simulink model "sim_sistema_2"  (Simulink 7.5)
settings: Solver=ode3  StartTime=0.0  StopTime=10  FixedStep=1e-4  RelTol=1e-3
values from neighbouring files (symbols this model uses):
  K = acker(sis.a,sis.b,J)    [sistema_2.m]    (also in sistema_2_observador.m)
  sis = ss(sis)    [sistema_2.m]    (also in sistema_2_observador.m)
settings Model: Creator=taniel.franklin  LastModifiedBy=taniel.franklin

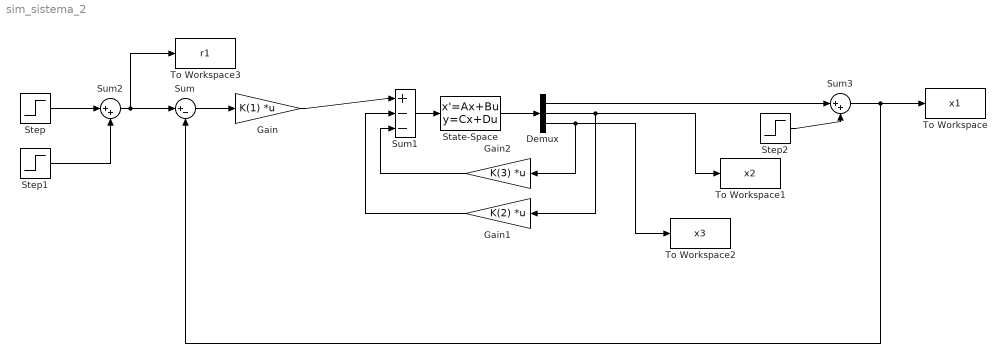
== system sim_sistema_2 ==
  Demux : Demux  Outputs=3
  Gain : Gain  Gain=K(1)  Multiplication=Matrix(K*u)  ParameterDataType=fixdt(1, 16)  ParameterScaling=2^0  OutDataType=fixdt(1, 16)  OutScaling=2^0
  Gain1 : Gain  Gain=K(2)  Multiplication=Matrix(K*u)  ParameterDataType=fixdt(1, 16)  ParameterScaling=2^0  OutDataType=fixdt(1, 16)  OutScaling=2^0
  Gain2 : Gain  Gain=K(3)  Multiplication=Matrix(K*u)  ParameterDataType=fixdt(1, 16)  ParameterScaling=2^0  OutDataType=fixdt(1, 16)  OutScaling=2^0
  State-Space : StateSpace  A=sis.A  B=sis.B  C=eye(3)  D=[0;0;0]
  Step : Step  Time=0.2  SampleTime=0
  Step1 : Step  Time=3  SampleTime=0
  Step2 : Step  Time=6  After=-1  SampleTime=0
  Sum : Sum  Inputs=|+-  OutDataType=fixdt(1, 16)  OutScaling=2^0
  Sum1 : Sum  Inputs=|+--  OutDataType=fixdt(1, 16)  OutScaling=2^0
  Sum2 : Sum  Inputs=|++  OutDataType=fixdt(1, 16)  OutScaling=2^0
  Sum3 : Sum  Inputs=|++  OutDataType=fixdt(1, 16)  OutScaling=2^0
  To Workspace : ToWorkspace  VariableName=x1  SampleTime=-1  SaveFormat=Structure With Time
  To Workspace1 : ToWorkspace  VariableName=x2  SampleTime=-1  SaveFormat=Structure With Time
  To Workspace2 : ToWorkspace  VariableName=x3  SampleTime=-1  SaveFormat=Structure With Time
  To Workspace3 : ToWorkspace  VariableName=r1  SampleTime=-1  SaveFormat=Structure With Time
  wires:
  State-Space/1 -> Demux/1
  Demux/2 -> To Workspace1/1, Gain1/1
  Demux/3 -> To Workspace2/1, Gain2/1
  Gain/1 -> Sum1/1
  Sum/1 -> Gain/1
  Sum1/1 -> State-Space/1
  Gain1/1 -> Sum1/2
  Step/1 -> Sum2/1
  Step1/1 -> Sum2/2
  Sum2/1 -> Sum/1, To Workspace3/1
  Gain2/1 -> Sum1/3
  Step2/1 -> Sum3/2
  Demux/1 -> Sum3/1
  Sum3/1 -> To Workspace/1, Sum/2
